simulink model "quad_CAD_asgsm"  (R2024a)
settings: Solver=ode4  StartTime=0.0  StopTime=60  FixedStep=0.01  RelTol=1e-3
undefined symbols (not defined in the file): F, Light, MIL, smiData, X, Y, Z
libraries: sm_lib x221, nesl_utility x22, dspobslib x9, sharedtransform x6, simulink x3, aerolibutil x2, matrix_library x1, sharedutil x1, robotcorelib x1, aerolibwind2 x1
(part 3 of 7)

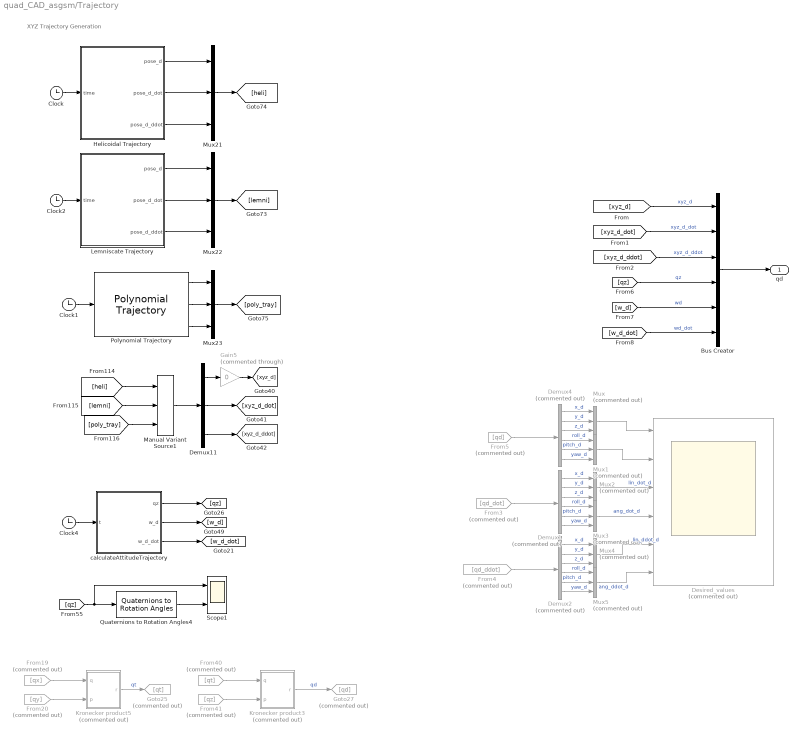
== system quad_CAD_asgsm/Trajectory ==
  note: XYZ Trajectory Generation
  Bus Creator : BusCreator  Inputs=6
  Clock{,1..2,4} (4 alike) : Clock
  Demux1 : Demux  Commented=on  Outputs=6
  Demux11 : Demux  Outputs=3
  Demux2 : Demux  Commented=on  Outputs=6
  Demux4 : Demux  Commented=on  Outputs=6
  Desired_values : Scope  Commented=on  NumInputPorts=6
  From19 : From  Commented=on  GotoTag=qx
  From20 : From  Commented=on  GotoTag=qy
  From3 : From  Commented=on  GotoTag=qd_dot
  From4 : From  Commented=on  GotoTag=qd_ddot
  From40 : From  Commented=on  GotoTag=qt
  From41 : From  Commented=on  GotoTag=qz
  From5 : From  Commented=on  GotoTag=qd
  Gain5 : Gain  Commented=through  Gain=0
  Goto25 : Goto  Commented=on  GotoTag=qt
  Goto27 : Goto  Commented=on  GotoTag=qd
  Helicoidal Trajectory : MATLAB Function  TreatAsAtomicUnit=on
  Kronecker product3 : Subsystem  Commented=on
  Kronecker product5 : Subsystem  Commented=on
  Lemniscate Trajectory : MATLAB Function  TreatAsAtomicUnit=on
  Manual Variant Source1 : simulink/Signal Routing/Manual Variant Source  NumChoices=3  LabelModeActiveChoice=V_3
  Mux{,1..5} (6 alike) : Mux  Commented=on  Inputs=3
  Mux21 : Mux  Inputs=3
  Mux22 : Mux  Inputs=3
  Mux23 : Mux  Inputs=3
  Polynomial Trajectory : robotcorelib/Polynomial Trajectory  WaypointSource=Internal  Waypoints=zeros(3, 6)  TimePoints=[ 0, 12, 24, 36, 48, 60]  TimeInterval=[ 1, 4 ]  Method=Cubic Polynomial  ParameterSource=Internal  VelocityBoundaryCondition=zeros( 3, 6)  AccelerationBoundaryCondition=zeros( 2, 5 )  SimulateUsing=Interpreted execution
  Quaternions to Rotation Angles4 : sharedtransform/Quaternions to Rotation Angles  rotationOrder=ZYX  aMode=aMode
  Scope1 : Scope  NumInputPorts=2
  calculateAttitudeTrajectory : MATLAB Function  TreatAsAtomicUnit=on
  qd : Outport
  wires:
  Demux4/6 -> Mux1/3  "yaw_d"
  Helicoidal Trajectory/2(pose_d_dot) -> Mux21/2
  Demux2/5 -> Mux5/2  "pitch_d"
  Demux4/1 -> Mux/1  "x_d"
  From3/1 -> Demux1/1
  calculateAttitudeTrajectory/3(w_d_dot) -> [w_d_dot]
  [xyz_d_dot] -> Bus Creator/2  "xyz_d_dot"
  Lemniscate Trajectory/1(pose_d) -> Mux22/1
  Bus Creator/1 -> qd/1
  Kronecker product5/1(r) -> Goto25/1  "qt"
  Demux2/6 -> Mux5/3  "yaw_d"
  From20/1 -> Kronecker product5/2(p)
  Demux1/6 -> Mux3/3  "yaw_d"
  Mux1/1 -> Desired_values/2
  From41/1 -> Kronecker product3/2(p)
  From40/1 -> Kronecker product3/1(q)
  Demux11/2 -> [xyz_d_dot]
  Lemniscate Trajectory/3(pose_d_ddot) -> Mux22/3
  Mux/1 -> Desired_values/1
  Lemniscate Trajectory/2(pose_d_dot) -> Mux22/2
  [lemni] -> Manual Variant Source1/2
  Gain5/1 -> [xyz_d]
  From19/1 -> Kronecker product5/1(q)
  Demux4/2 -> Mux/2  "y_d"
  Mux2/1 -> Desired_values/3  "lin_dot_d"
  [xyz_d] -> Bus Creator/1  "xyz_d"
  Demux4/5 -> Mux1/2  "pitch_d"
  Polynomial Trajectory/2 -> Mux23/2
  Helicoidal Trajectory/3(pose_d_ddot) -> Mux21/3
  [heli] -> Manual Variant Source1/1
  [w_d] -> Bus Creator/5  "wd"
  Polynomial Trajectory/3 -> Mux23/3
  Clock/1 -> Helicoidal Trajectory/1(time)
  calculateAttitudeTrajectory/2(w_d) -> [w_d]
  Demux2/1 -> Mux4/1  "x_d"
  [qz] -> Bus Creator/4  "qz"
  Clock4/1 -> calculateAttitudeTrajectory/1(t)
  Mux22/1 -> [lemni]
  [qz] -> Scope1/1, Quaternions to Rotation Angles4/1
  Clock2/1 -> Lemniscate Trajectory/1(time)
  Polynomial Trajectory/1 -> Mux23/1
  calculateAttitudeTrajectory/1(qz) -> [qz]
  Mux21/1 -> [heli]
  Demux4/3 -> Mux/3  "z_d"
  Demux2/4 -> Mux5/1  "roll_d"
  Mux3/1 -> Desired_values/4  "ang_dot_d"
  Mux4/1 -> Desired_values/5  "lin_ddot_d"
  Demux4/4 -> Mux1/1  "roll_d"
  Demux1/1 -> Mux2/1  "x_d"
  Demux1/2 -> Mux2/2  "y_d"
  [xyz_d_ddot] -> Bus Creator/3  "xyz_d_ddot"
  Demux2/3 -> Mux4/3  "z_d"
  From4/1 -> Demux2/1
  [w_d_dot] -> Bus Creator/6  "wd_dot"
  Mux5/1 -> Desired_values/6  "ang_ddot_d"
  Demux11/1 -> Gain5/1
  [poly_tray] -> Manual Variant Source1/3
  From5/1 -> Demux4/1
  Clock1/1 -> Polynomial Trajectory/1
  Kronecker product3/1(r) -> Goto27/1  "qd"
  Quaternions to Rotation Angles4/1 -> Scope1/2
  Helicoidal Trajectory/1(pose_d) -> Mux21/1
  Mux23/1 -> [poly_tray]
  Demux1/3 -> Mux2/3  "z_d"
  Demux1/4 -> Mux3/1  "roll_d"
  Manual Variant Source1/1 -> Demux11/1
  Demux11/3 -> [xyz_d_ddot]
  Demux1/5 -> Mux3/2  "pitch_d"
  Demux2/2 -> Mux4/2  "y_d"

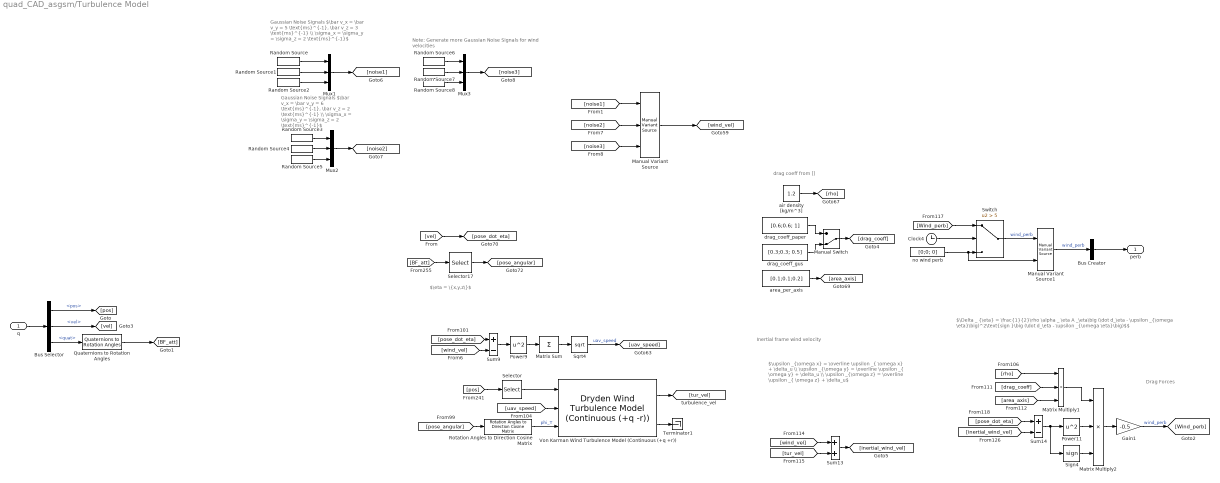
== system quad_CAD_asgsm/Turbulence Model ==
  note: Note: Generate more Gaussian Noise Signals
      | for wind velocities
  note: $\Delta _ {\eta} = \frac{1}{2}\rho \alpha _ \eta A _\eta\big (\dot d_\eta - \upsilon _{\omega \eta}\big)^2\text{sign }\big (\dot d_\eta - \upsilon _{\omega \eta}\big)$$
  note: $\upsilon _{\omega x} = \overline \upsilon _{ \omega x} + \delta_u \\ \upsilon _{\omega y} = \overline \upsilon _{ \omega y} + \delta_u \\ \upsilon _{\omega z} = \overline \upsilon _{ \omega z} + \delta_u$
  note: drag coeff from []
  note: Drag Forces
  note: Inertial frame wind velocity
  note: $\eta = \{x,y,z\}$
  note: Gaussian Noise Signals
      | $\bar v_x = \bar v_y = 6 \text{ms}^{-1}, \bar v_z = 2 \text{ms}^{-1} \\ \sigma_x = \sigma_y = \sigma_z = 2 \text{ms}^{-1}$
  note: Gaussian Noise Signals
      | $\bar v_x = \bar v_y = 5 \text{ms}^{-1}, \bar v_z = 3 \text{ms}^{-1} \\ \sigma_x = \sigma_y = \sigma_z = 2 \text{ms}^{-1}$
  q : Inport
  Bus Creator : BusCreator  Inputs=1
  Bus Selector : BusSelector  OutputSignals=pos,vel,quat
  Clock4 : Clock
  Gain1 : Gain  Gain=-0.5
  Manual Variant Source : simulink/Signal Routing/Manual Variant Source  NumChoices=3  LabelModeActiveChoice=V_1
  Manual Variant Source1 : simulink/Signal Routing/Manual Variant Source  NumChoices=2  LabelModeActiveChoice=V_1
  Manual Switch : ManualSwitch  CurrentSetting=0
  Matrix Sum : Sum  Inputs=+
  Matrix Multiply1 : Product  Inputs=3
  Matrix Multiply2 : Product  Inputs=3
  Mux1 : Mux  Inputs=3
  Mux2 : Mux  Inputs=3
  Mux3 : Mux  Inputs=3
  Power11 : Math  Operator=square
  Power9 : Math  Operator=square
  Quaternions to Rotation Angles : sharedtransform/Quaternions to Rotation Angles  rotationOrder=ZYX  aMode=aMode
  Random Source : dspobslib/Random Source  SrcType=Gaussian  NormMethod=Ziggurat  CltLength=12  MinVal=0  MaxVal=1  MeanVal=5  VarVal=2  RepMode=Not repeatable  rawSeed=1  IsInherit=off  SampMode=Discrete  SampTime=1  SampFrame=1  DataType=Double  OutComplex=Real  OutputFrames=off
  Random Source1 : dspobslib/Random Source  SrcType=Gaussian  NormMethod=Ziggurat  CltLength=12  MinVal=0  MaxVal=1  MeanVal=5  VarVal=2  RepMode=Not repeatable  rawSeed=1  IsInherit=off  SampMode=Discrete  SampTime=1  SampFrame=1  DataType=Double  OutComplex=Real  OutputFrames=off
  Random Source2 : dspobslib/Random Source  SrcType=Gaussian  NormMethod=Ziggurat  CltLength=12  MinVal=0  MaxVal=1  MeanVal=3  VarVal=2  RepMode=Not repeatable  rawSeed=1  IsInherit=off  SampMode=Discrete  SampTime=1  SampFrame=1  DataType=Double  OutComplex=Real  OutputFrames=off
  Random Source{3..4,6..7} (4 alike) : dspobslib/Random Source  SrcType=Gaussian  NormMethod=Ziggurat  CltLength=12  MinVal=0  MaxVal=1  MeanVal=6  VarVal=2  RepMode=Not repeatable  rawSeed=1  IsInherit=off  SampMode=Discrete  SampTime=1  SampFrame=1  DataType=Double  OutComplex=Real  OutputFrames=off
  Random Source5 : dspobslib/Random Source  SrcType=Gaussian  NormMethod=Ziggurat  CltLength=12  MinVal=0  MaxVal=1  MeanVal=2  VarVal=2  RepMode=Not repeatable  rawSeed=1  IsInherit=off  SampMode=Discrete  SampTime=1  SampFrame=1  DataType=Double  OutComplex=Real  OutputFrames=off
  Random Source8 : dspobslib/Random Source  SrcType=Gaussian  NormMethod=Ziggurat  CltLength=12  MinVal=0  MaxVal=1  MeanVal=2  VarVal=2  RepMode=Not repeatable  rawSeed=1  IsInherit=off  SampMode=Discrete  SampTime=1  SampFrame=1  DataType=Double  OutComplex=Real  OutputFrames=off
  Rotation Angles to Direction Cosine Matrix : sharedtransform/Rotation Angles to Direction Cosine Matrix  rotationOrder=XYZ  aMode=aMode
  Selector : Selector  InputPortWidth=3  IndexOptions=Index vector (dialog)  Indices=[3]  OutputSizes=1
  Selector17 : Selector  InputPortWidth=3  IndexOptions=Index vector (dialog)  Indices=[3 2 1]  OutputSizes=1
  Sign4 : Signum
  Sqrt4 : Sqrt
  Sum13 : Sum
  Sum14 : Sum  Inputs=+-
  Sum9 : Sum  Inputs=+-
  Switch : Switch  Criteria=u2 > Threshold  Threshold=5  SaturateOnIntegerOverflow=off  InputSameDT=off
  Terminator1 : Terminator
  Von Karman Wind Turbulence Model (Continuous (+q +r)) : aerolibwind2/Dryden Wind Turbulence Model  (Continuous (+q -r))  units=Metric (MKS)  spec=MIL-F-8785C  model=Continuous Von Karman (+q -r)  W20=15  Wdeg=0  TurbProb=10^-2 - Light  L_high=762  Wingspan=10  ts=0.1  Seed=[23341 23342 23343 23344]  T_on=on
      settings: LibrarySourceBlock=|
      | aerolibwind2/Von Karman Wind Turbulence Model
      | (Continuous (+q +r))
  air density [kg/m^3] : Constant  Value=1.2
  area_per_axis : Constant  Value=[0.1;0.1;0.2]
  drag_coeff_gus : Constant  Value=[0.3;0.3; 0.5]
  drag_coeff_paper : Constant  Value=[0.6;0.6; 1]
  no wind perb : Constant  Value=[0;0; 0]
  perb : Outport
  wires:
  [rho] -> Matrix Multiply1/1
  [drag_coeff] -> Matrix Multiply1/2
  Von Karman Wind Turbulence Model (Continuous (+q +r))/2 -> Terminator1/1
  area_per_axis/1 -> [area_axis]
  [pose_dot_eta] -> Sum14/1
  Von Karman Wind Turbulence Model (Continuous (+q +r))/1 -> [tur_vel]
  [wind_vel] -> Sum9/2
  Selector17/1 -> [pose_angular]
  Matrix Multiply1/1 -> Matrix Multiply2/1
  Sign4/1 -> Matrix Multiply2/3
  [uav_speed] -> Von Karman Wind Turbulence Model (Continuous (+q +r))/2
  Power9/1 -> Matrix Sum/1
  Sqrt4/1 -> [uav_speed]  "uav_speed"
  Gain1/1 -> [Wind_perb]  "wind_perb"
  Sum9/1 -> Power9/1
  air density [kg/m^3]/1 -> [rho]
  Clock4/1 -> Switch/2
  [pose_dot_eta] -> Sum9/1
  Rotation Angles to Direction Cosine Matrix/1 -> Von Karman Wind Turbulence Model (Continuous (+q +r))/3  "phi_T"
  [tur_vel] -> Sum13/2
  Sum14/1 -> Sign4/1, Power11/1
  no wind perb/1 -> Manual Variant Source1/2, Switch/3
  drag_coeff_gus/1 -> Manual Switch/2
  Switch/1 -> Manual Variant Source1/1  "wind_perb"
  [area_axis] -> Matrix Multiply1/3
  Manual Switch/1 -> [drag_coeff]
  Selector/1 -> Von Karman Wind Turbulence Model (Continuous (+q +r))/1
  [pose_angular] -> Rotation Angles to Direction Cosine Matrix/1
  [inertial_wind_vel] -> Sum14/2
  Matrix Multiply2/1 -> Gain1/1
  drag_coeff_paper/1 -> Manual Switch/1
  Power11/1 -> Matrix Multiply2/2
  Matrix Sum/1 -> Sqrt4/1
  Sum13/1 -> [inertial_wind_vel]
  [Wind_perb] -> Switch/1
  [wind_vel] -> Sum13/1
  Bus Creator/1 -> perb/1
  [BF_att] -> Selector17/1
  [pos] -> Selector/1
  q/1 -> Bus Selector/1
  Bus Selector/1 -> [pos]  "<pos>"
  Bus Selector/3 -> Quaternions to Rotation Angles/1  "<quat>"
  Bus Selector/2 -> [vel]  "<vel>"
  [vel] -> [pose_dot_eta]
  Mux2/1 -> [noise2]
  Random Source5/1 -> Mux2/3
  Random Source/1 -> Mux1/1
  Mux1/1 -> [noise1]
  Random Source2/1 -> Mux1/3
  Random Source4/1 -> Mux2/2
  Random Source3/1 -> Mux2/1
  [noise2] -> Manual Variant Source/2
  Manual Variant Source/1 -> [wind_vel]
  Random Source1/1 -> Mux1/2
  [noise1] -> Manual Variant Source/1
  [noise3] -> Manual Variant Source/3
  Mux3/1 -> [noise3]
  Random Source7/1 -> Mux3/2
  Random Source6/1 -> Mux3/1
  Random Source8/1 -> Mux3/3
  Manual Variant Source1/1 -> Bus Creator/1  "wind_perb"
  Quaternions to Rotation Angles/1 -> [BF_att]

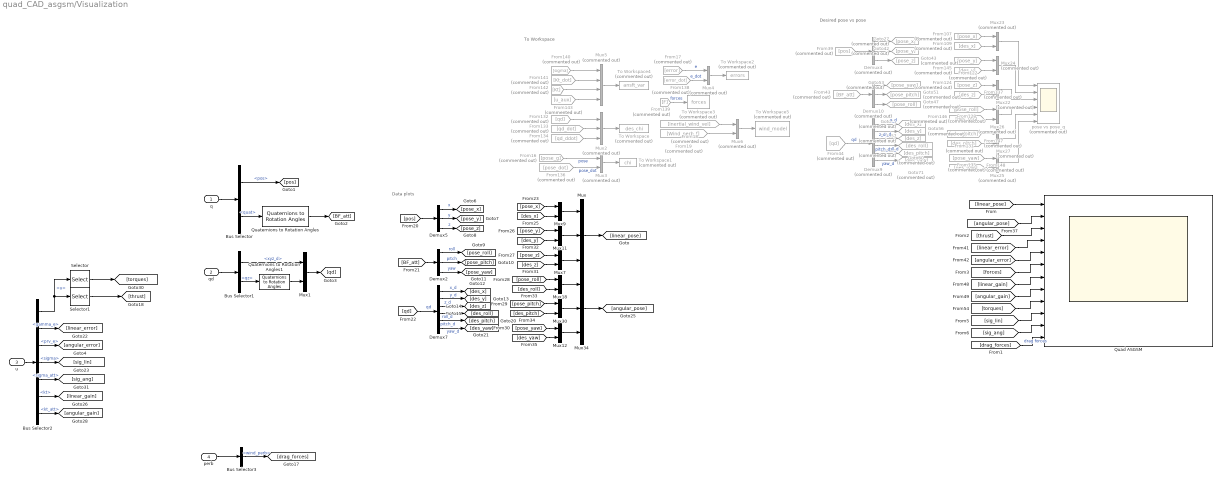
== system quad_CAD_asgsm/Visualization ==
  note: Desired pose vs pose
  note: Data plots
  note: To Workspace
  q : Inport
  qd : Inport  Port=2
  u : Inport  Port=3
  perb : Inport  Port=4
  Bus Selector : BusSelector  OutputSignals=pos,quat
  Bus Selector1 : BusSelector  OutputSignals=xyz_d,qz
  Bus Selector2 : BusSelector  OutputSignals=u,gamma_e,prv_e,sigma,sigma_att,kt,kt_att
  Bus Selector3 : BusSelector  OutputSignals=wind_perb
  Demux10 : Demux  Commented=on  Outputs=3
  Demux2 : Demux  Outputs=3
  Demux4 : Demux  Commented=on  Outputs=3
  Demux5 : Demux  Outputs=3
  Demux7 : Demux  Outputs=6
  Demux9 : Demux  Commented=on  Outputs=6
  From107 : From  Commented=on  GotoTag=pose_x
  From109 : From  Commented=on  GotoTag=des_x
  From122 : From  Commented=on  GotoTag=pose_y
  From124 : From  Commented=on  GotoTag=pose_z
  From128 : From  Commented=on  GotoTag=pose_roll
  From131 : From  Commented=on  GotoTag=pose_pitch
  From132 : From  Commented=on  GotoTag=qd
  From133 : From  Commented=on  GotoTag=qd_dot
  From134 : From  Commented=on  GotoTag=qd_ddot
  From135 : From  Commented=on  GotoTag=pose_yaw
  From136 : From  Commented=on  GotoTag=pose_dot
  From137 : From  Commented=on  GotoTag=des_z
  From138 : From  Commented=on  GotoTag=error_dot
  From139 : From  Commented=on  GotoTag=F
  From140 : From  Commented=on  GotoTag=sigma
  From141 : From  Commented=on  GotoTag=Kt_dot
  From142 : From  Commented=on  GotoTag=Kt
  From143 : From  Commented=on  GotoTag=u_aux
  From145 : From  Commented=on  GotoTag=des_y
  From146 : From  Commented=on  GotoTag=des_roll
  From147 : From  Commented=on  GotoTag=des_pitch
  From148 : From  Commented=on  GotoTag=des_yaw
  From16 : From  Commented=on  GotoTag=pose_g
  From17 : From  Commented=on  GotoTag=error
  From18 : From  Commented=on  GotoTag=inertial_wind_vel
  From19 : From  Commented=on  GotoTag=Wind_perb_f  TagVisibility=global
  From39 : From  Commented=on  GotoTag=pos
  From43 : From  Commented=on  GotoTag=BF_att
  From44 : From  Commented=on  GotoTag=qd
  Goto27 : Goto  Commented=on  GotoTag=pose_x
  Goto42 : Goto  Commented=on  GotoTag=pose_y
  Goto43 : Goto  Commented=on  GotoTag=pose_z
  Goto47 : Goto  Commented=on  GotoTag=pose_roll
  Goto51 : Goto  Commented=on  GotoTag=pose_pitch
  Goto53 : Goto  Commented=on  GotoTag=pose_yaw
  Goto55 : Goto  Commented=on  GotoTag=des_x
  Goto56 : Goto  Commented=on  GotoTag=des_y
  Goto57 : Goto  Commented=on  GotoTag=des_z
  Goto60 : Goto  Commented=on  GotoTag=des_roll
  Goto68 : Goto  Commented=on  GotoTag=des_pitch
  Goto71 : Goto  Commented=on  GotoTag=des_yaw
  Mux : Mux  Inputs=3
  Mux{1,7,9,11..12,18,30} (7 alike) : Mux  Inputs=2
  Mux2 : Mux  Commented=on  Inputs=3
  Mux{3..4,6,22..27} (9 alike) : Mux  Commented=on  Inputs=2
  Mux34 : Mux  Inputs=3
  Mux5 : Mux  Commented=on
  Quad ASGSM : Scope  NumInputPorts=12
  Quaternions to Rotation Angles : sharedtransform/Quaternions to Rotation Angles  rotationOrder=XYZ  aMode=aMode
  Quaternions to Rotation Angles1 : sharedtransform/Quaternions to Rotation Angles  rotationOrder=XYZ  aMode=aMode
  Selector : Selector  InputPortWidth=4  IndexOptions=Index vector (dialog)  Indices=[1:3]  OutputSizes=1
  Selector1 : Selector  InputPortWidth=4  IndexOptions=Index vector (dialog)  Indices=[4]  OutputSizes=1
  To Workspace : ToWorkspace  Commented=on  VariableName=des_chi  SaveFormat=Structure With Time  SampleTime=-1
  To Workspace1 : ToWorkspace  Commented=on  VariableName=chi  SaveFormat=Structure With Time  SampleTime=-1
  To Workspace2 : ToWorkspace  Commented=on  VariableName=errors  SaveFormat=Structure With Time  SampleTime=-1
  To Workspace3 : ToWorkspace  Commented=on  VariableName=forces  SaveFormat=Structure With Time  SampleTime=-1
  To Workspace4 : ToWorkspace  Commented=on  VariableName=ansft_var  SaveFormat=Structure With Time  SampleTime=-1
  To Workspace5 : ToWorkspace  Commented=on  VariableName=wind_model  SaveFormat=Structure With Time  SampleTime=-1
  pose vs pose_q : Scope  Commented=on  NumInputPorts=6
  wires:
  Mux/1 -> [linear_pose]
  Mux6/1 -> To Workspace5/1
  Mux9/1 -> Mux/1
  From128/1 -> Mux26/1
  Demux4/1 -> Goto27/1
  Demux7/5 -> [des_pitch]  "pitch_d"
  From135/1 -> Mux25/1
  [linear_error] -> Quad ASGSM/4
  [angular_error] -> Quad ASGSM/5
  From132/1 -> Mux2/1
  Mux11/1 -> Mux/2
  Demux4/3 -> Goto43/1
  Demux5/1 -> [pose_x]  "x"
  Demux10/1 -> Goto53/1
  Demux10/3 -> Goto47/1
  Mux3/1 -> To Workspace1/1
  Demux5/3 -> [pose_z]  "z"
  From148/1 -> Mux25/2
  Demux9/6 -> Goto71/1  "yaw_d"
  [BF_att] -> Demux2/1
  Mux23/1 -> pose vs pose_q/1
  Demux9/2 -> Goto56/1  "y_d"
  Demux7/2 -> [des_y]  "y_d"
  Demux5/2 -> [pose_y]  "y"
  From16/1 -> Mux3/1  "pose"
  [pose_pitch] -> Mux30/1
  [pose_y] -> Mux11/1
  From44/1 -> Demux9/1  "qd"
  Demux7/3 -> [des_z]  "z_d"
  [angular_gain] -> Quad ASGSM/8
  From133/1 -> Mux2/2
  [des_pitch] -> Mux30/2
  Mux5/1 -> To Workspace4/1
  [linear_gain] -> Quad ASGSM/7
  Mux2/1 -> To Workspace/1
  [des_roll] -> Mux18/2
  From43/1 -> Demux10/1
  Mux22/1 -> pose vs pose_q/3
  Mux26/1 -> pose vs pose_q/4
  Mux24/1 -> pose vs pose_q/2
  From109/1 -> Mux23/2
  Demux7/4 -> [des_roll]  "roll_d"
  Demux9/4 -> Goto60/1  "roll_d"
  From122/1 -> Mux24/1
  [des_yaw] -> Mux12/2
  From139/1 -> To Workspace3/1  "forces"
  [angular_pose] -> Quad ASGSM/2
  Demux9/3 -> Goto57/1  "z_d"
  From124/1 -> Mux22/1
  Demux7/1 -> [des_x]  "x_d"
  From138/1 -> Mux4/2  "e_dot"
  [pose_yaw] -> Mux12/1
  From39/1 -> Demux4/1
  From137/1 -> Mux22/2
  Mux12/1 -> Mux34/3
  From131/1 -> Mux27/1
  [des_x] -> Mux9/2
  [linear_pose] -> Quad ASGSM/1
  Demux9/1 -> Goto55/1  "x_d"
  [pos] -> Demux5/1
  From18/1 -> Mux6/1
  From141/1 -> Mux5/2
  Mux7/1 -> Mux/3
  From145/1 -> Mux24/2
  Demux9/5 -> Goto68/1  "pitch_d"
  From17/1 -> Mux4/1  "e"
  Mux34/1 -> [angular_pose]
  [pose_x] -> Mux9/1
  Demux10/2 -> Goto51/1
  [pose_roll] -> Mux18/1
  [pose_z] -> Mux7/1
  Mux30/1 -> Mux34/2
  [des_y] -> Mux11/2
  Demux7/6 -> [des_yaw]  "yaw_d"
  Mux4/1 -> To Workspace2/1
  From19/1 -> Mux6/2
  From134/1 -> Mux2/3
  Mux18/1 -> Mux34/1
  Demux4/2 -> Goto42/1
  [qd] -> Demux7/1  "qd"
  From143/1 -> Mux5/4
  From146/1 -> Mux26/2
  Mux27/1 -> pose vs pose_q/5
  [des_z] -> Mux7/2
  From147/1 -> Mux27/2
  From142/1 -> Mux5/3
  From140/1 -> Mux5/1
  From136/1 -> Mux3/2  "pose_dot"
  From107/1 -> Mux23/1
  Mux25/1 -> pose vs pose_q/6
  q/1 -> Bus Selector/1
  Bus Selector/1 -> [pos]  "<pos>"
  Bus Selector/2 -> Quaternions to Rotation Angles/1  "<quat>"
  qd/1 -> Bus Selector1/1
  Bus Selector1/1 -> Mux1/1  "<xyz_d>"
  u/1 -> Bus Selector2/1
  perb/1 -> Bus Selector3/1
  Bus Selector3/1 -> [drag_forces]  "<wind_perb>"
  [thrust] -> Quad ASGSM/3
  [forces] -> Quad ASGSM/6
  [torques] -> Quad ASGSM/9
  [drag_forces] -> Quad ASGSM/12  "drag forces"
  [sig_lin] -> Quad ASGSM/10
  [sig_ang] -> Quad ASGSM/11
  Demux2/2 -> [pose_pitch]  "pitch"
  Demux2/3 -> [pose_yaw]  "yaw"
  Demux2/1 -> [pose_roll]  "roll"
  Quaternions to Rotation Angles/1 -> [BF_att]
  Bus Selector2/1 -> Selector1/1, Selector/1  "<u>"
  Selector/1 -> [torques]
  Selector1/1 -> [thrust]
  Bus Selector2/5 -> [sig_ang]  "<sigma_att>"
  Bus Selector2/7 -> [angular_gain]  "<kt_att>"
  Bus Selector2/6 -> [linear_gain]  "<kt>"
  Bus Selector2/4 -> [sig_lin]  "<sigma>"
  Bus Selector2/3 -> [angular_error]  "<prv_e>"
  Bus Selector2/2 -> [linear_error]  "<gamma_e>"
  Bus Selector1/2 -> Quaternions to Rotation Angles1/1  "<qz>"
  Quaternions to Rotation Angles1/1 -> Mux1/2
  Mux1/1 -> [qd]

== system quad_CAD_asgsm/Controller/Attitude_Alignment ==
  nu : Inport
  nz : Inport  Port=2
  Scope : Scope  NumInputPorts=2
  attitude_alignment : MATLAB Function  TreatAsAtomicUnit=on
  qt : Outport
  wires:
  attitude_alignment/1(qt) -> qt/1
  nz/1 -> attitude_alignment/2("nz ")
  nu/1 -> attitude_alignment/1(u)
  attitude_alignment/2(nz) -> Scope/1
  attitude_alignment/3(nu) -> Scope/2

== system quad_CAD_asgsm/Controller/Kronecker product3 ==
  q : Inport
  p : Inport  Port=2
  Kronecker_product : MATLAB Function  TreatAsAtomicUnit=on
  r : Outport
  wires:
  q/1 -> Kronecker_product/1(q)
  p/1 -> Kronecker_product/2(p)
  Kronecker_product/1(r) -> r/1

== system quad_CAD_asgsm/Controller/Kronecker product4 ==
  q : Inport
  p : Inport  Port=2
  Kronecker_product : MATLAB Function  TreatAsAtomicUnit=on
  r : Outport
  wires:
  q/1 -> Kronecker_product/1(q)
  p/1 -> Kronecker_product/2(p)
  Kronecker_product/1(r) -> r/1

== system quad_CAD_asgsm/Controller/Subsystem1 ==
  q : Inport
  MATLAB Function : MATLAB Function  TreatAsAtomicUnit=on
  lnq : Outport
  wires:
  MATLAB Function/1(lnq) -> lnq/1
  q/1 -> MATLAB Function/1(q)

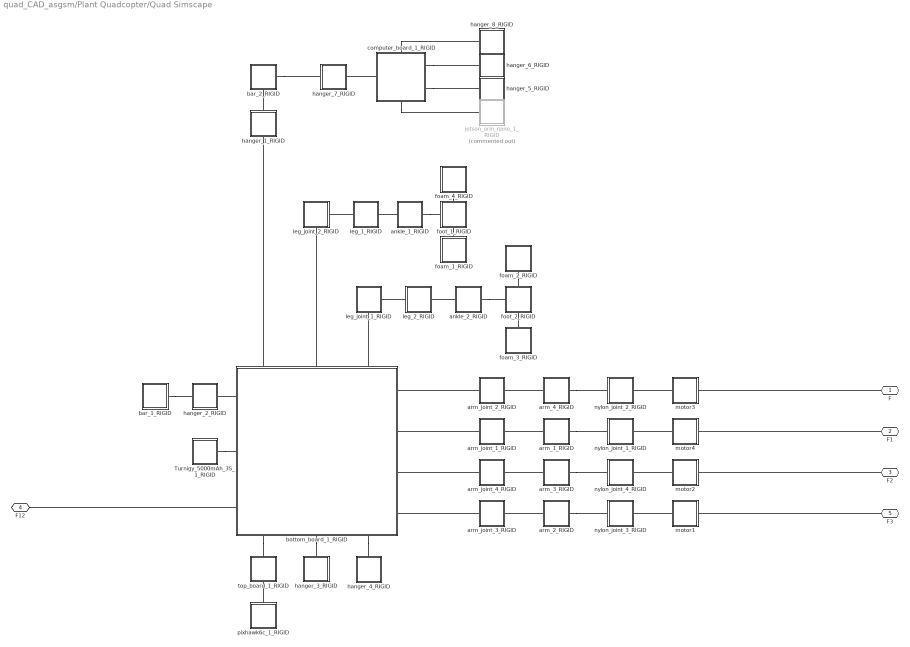
== system quad_CAD_asgsm/Plant Quadcopter/Quad Simscape ==
  Turnigy_5000mAh_3S_1_RIGID : Subsystem
  ankle_1_RIGID : Subsystem
  ankle_2_RIGID : Subsystem
  arm_1_RIGID : Subsystem
  arm_2_RIGID : Subsystem
  arm_3_RIGID : Subsystem
  arm_4_RIGID : Subsystem
  arm_joint_1_RIGID : Subsystem
  arm_joint_2_RIGID : Subsystem
  arm_joint_3_RIGID : Subsystem
  arm_joint_4_RIGID : Subsystem
  bar_1_RIGID : Subsystem
  bar_2_RIGID : Subsystem
      settings: PortSchema="{\"entries\":[{\"content\":{\"sides\":[{\"content\":{},\"type\":\"ConnectorPlacement.EquallySpacedRectSide\",\"uuid\":\"e4c68bcb-f3fe-4aba-8bbb-748bf6c2ba1e\"},{\"content\":{\"connectorIds\":[\"RConn1\"],\"side\":\"RIGHT\"},\"type\":\"ConnectorPlacement.EquallySpacedRectSide\",\"uuid\":\"1338b84e-cb3b-43ed-b934-4b64495642c6\"},{\"content\":{\"side\":\"TOP\"},\"type\":\"ConnectorPlacement.EquallySpacedRectSide\",\"uuid\":\"c07eb51d-104f-4d2f-bffb-19c5e8e904cd\"},{\"content\":{\"connectorIds\":[\"RConn2\"],\"side\":\"BOTTOM\"},\"type\":\"ConnectorPlacement.EquallySpacedRectSide\",\"uuid\":\"9f3520f2-c2cf-4d2b-85d9-f0e92fcce62d\"}]},\"type\":\"ConnectorPlacement.EquallySpacedConnector\",\"uuid\":\"66267511-5957-447d-be6d-58b2f28344a3\"}],\"packageUris\":[\"http://schema.mathworks.com/mf0/Connector/R2020b\"],\"version\":\"1.0\"}"
  bottom_board_1_RIGID : Subsystem
      settings: PortSchema="{\"entries\":[{\"content\":{\"sides\":[{\"content\":{\"connectorIds\":[\"LConn1\",\"LConn2\",\"LConn3\"]},\"type\":\"ConnectorPlacement.EquallySpacedRectSide\",\"uuid\":\"9aceb689-13c3-4410-a12b-a205fc5c5e29\"},{\"content\":{\"connectorIds\":[\"RConn1\",\"RConn2\",\"RConn3\",\"RConn4\"],\"side\":\"RIGHT\"},\"type\":\"ConnectorPlacement.EquallySpacedRectSide\",\"uuid\":\"62657ca3-c014-471d-8baa-8f5757c474c2\"},{\"content\":{\"connectorIds\":[\"LConn4\",\"LConn5\",\"LConn6\"],\"side\":\"TOP\"},\"type\":\"ConnectorPlacement.EquallySpacedRectSide\",\"uuid\":\"f572a818-8233-41db-820d-2371a42ad6c7\"},{\"content\":{\"connectorIds\":[\"RConn5\",\"RConn6\",\"RConn7\"],\"side\":\"BOTTOM\"},\"type\":\"ConnectorPlacement.EquallySpacedRectSide\",\"uuid\":\"f4e3c856-449b-45f8-8e8a-d1faf7fe0ed6\"}]},\"type\":\"ConnectorPlacement.EquallySpacedConnector\",\"uuid\":\"18325c75-42ae-41d5-ba8b-a65f9cc18b57\"}],\"packageUris\":[\"http://schema.mathworks.com/mf0/Connector/R2020b\"],\"version\":\"1.0\"}"
  computer_board_1_RIGID : Subsystem
      settings: PortSchema="{\"entries\":[{\"content\":{\"sides\":[{\"content\":{\"connectorIds\":[\"LConn1\"]},\"type\":\"ConnectorPlacement.EquallySpacedRectSide\",\"uuid\":\"45520a5c-9755-44f8-961d-1edc3bf3f9b3\"},{\"content\":{\"connectorIds\":[\"RConn1\",\"RConn2\"],\"side\":\"RIGHT\"},\"type\":\"ConnectorPlacement.EquallySpacedRectSide\",\"uuid\":\"004a0d01-52c5-40e4-bd02-7a89b4d4e543\"},{\"content\":{\"connectorIds\":[\"LConn2\"],\"side\":\"TOP\"},\"type\":\"ConnectorPlacement.EquallySpacedRectSide\",\"uuid\":\"74e8819f-1d4d-4a14-976c-d3b18c4e091d\"},{\"content\":{\"connectorIds\":[\"RConn3\"],\"side\":\"BOTTOM\"},\"type\":\"ConnectorPlacement.EquallySpacedRectSide\",\"uuid\":\"f917d1f0-d232-4281-b426-7e15d7693ef0\"}]},\"type\":\"ConnectorPlacement.EquallySpacedConnector\",\"uuid\":\"e479e9d8-600b-48d5-99b2-6391ef29c8cc\"}],\"packageUris\":[\"http://schema.mathworks.com/mf0/Connector/R2020b\"],\"version\":\"1.0\"}"
  foam_1_RIGID : Subsystem
      settings: PortSchema="{\"entries\":[{\"content\":{\"sides\":[{\"content\":{},\"type\":\"ConnectorPlacement.EquallySpacedRectSide\",\"uuid\":\"7acb360a-1230-4e27-92b8-6b3184352f22\"},{\"content\":{\"side\":\"RIGHT\"},\"type\":\"ConnectorPlacement.EquallySpacedRectSide\",\"uuid\":\"8c89d56c-1eb2-4c7c-8666-e0d9ca480c9b\"},{\"content\":{\"connectorIds\":[\"LConn1\"],\"side\":\"TOP\"},\"type\":\"ConnectorPlacement.EquallySpacedRectSide\",\"uuid\":\"50379f80-a646-4b72-9568-e30937a88a17\"}]},\"type\":\"ConnectorPlacement.EquallySpacedConnector\",\"uuid\":\"0fd64392-f5bf-42bb-9262-b488cfdbbdbf\"}],\"packageUris\":[\"http://schema.mathworks.com/mf0/Connector/R2020b\"],\"version\":\"1.0\"}"
  foam_2_RIGID : Subsystem
      settings: PortSchema="{\"entries\":[{\"content\":{\"sides\":[{\"content\":{},\"type\":\"ConnectorPlacement.EquallySpacedRectSide\",\"uuid\":\"7acb360a-1230-4e27-92b8-6b3184352f22\"},{\"content\":{\"side\":\"RIGHT\"},\"type\":\"ConnectorPlacement.EquallySpacedRectSide\",\"uuid\":\"8c89d56c-1eb2-4c7c-8666-e0d9ca480c9b\"},{\"content\":{\"side\":\"TOP\"},\"type\":\"ConnectorPlacement.EquallySpacedRectSide\",\"uuid\":\"50379f80-a646-4b72-9568-e30937a88a17\"},{\"content\":{\"connectorIds\":[\"RConn1\"],\"side\":\"BOTTOM\"},\"type\":\"ConnectorPlacement.EquallySpacedRectSide\",\"uuid\":\"d189d42a-5809-41f4-8819-94bfeb6d4069\"}]},\"type\":\"ConnectorPlacement.EquallySpacedConnector\",\"uuid\":\"0fd64392-f5bf-42bb-9262-b488cfdbbdbf\"}],\"packageUris\":[\"http://schema.mathworks.com/mf0/Connector/R2020b\"],\"version\":\"1.0\"}"
  foam_3_RIGID : Subsystem
      settings: PortSchema="{\"entries\":[{\"content\":{\"sides\":[{\"content\":{},\"type\":\"ConnectorPlacement.EquallySpacedRectSide\",\"uuid\":\"7acb360a-1230-4e27-92b8-6b3184352f22\"},{\"content\":{\"side\":\"RIGHT\"},\"type\":\"ConnectorPlacement.EquallySpacedRectSide\",\"uuid\":\"8c89d56c-1eb2-4c7c-8666-e0d9ca480c9b\"},{\"content\":{\"connectorIds\":[\"LConn1\"],\"side\":\"TOP\"},\"type\":\"ConnectorPlacement.EquallySpacedRectSide\",\"uuid\":\"50379f80-a646-4b72-9568-e30937a88a17\"}]},\"type\":\"ConnectorPlacement.EquallySpacedConnector\",\"uuid\":\"0fd64392-f5bf-42bb-9262-b488cfdbbdbf\"}],\"packageUris\":[\"http://schema.mathworks.com/mf0/Connector/R2020b\"],\"version\":\"1.0\"}"
  foam_4_RIGID : Subsystem
      settings: PortSchema="{\"entries\":[{\"content\":{\"sides\":[{\"content\":{},\"type\":\"ConnectorPlacement.EquallySpacedRectSide\",\"uuid\":\"7acb360a-1230-4e27-92b8-6b3184352f22\"},{\"content\":{\"side\":\"RIGHT\"},\"type\":\"ConnectorPlacement.EquallySpacedRectSide\",\"uuid\":\"8c89d56c-1eb2-4c7c-8666-e0d9ca480c9b\"},{\"content\":{\"side\":\"TOP\"},\"type\":\"ConnectorPlacement.EquallySpacedRectSide\",\"uuid\":\"50379f80-a646-4b72-9568-e30937a88a17\"},{\"content\":{\"connectorIds\":[\"RConn1\"],\"side\":\"BOTTOM\"},\"type\":\"ConnectorPlacement.EquallySpacedRectSide\",\"uuid\":\"61179d7d-8587-4b45-83e9-ef742d015af7\"}]},\"type\":\"ConnectorPlacement.EquallySpacedConnector\",\"uuid\":\"0fd64392-f5bf-42bb-9262-b488cfdbbdbf\"}],\"packageUris\":[\"http://schema.mathworks.com/mf0/Connector/R2020b\"],\"version\":\"1.0\"}"
  foot_1_RIGID : Subsystem
      settings: PortSchema="{\"entries\":[{\"content\":{\"sides\":[{\"content\":{\"connectorIds\":[\"LConn1\"]},\"type\":\"ConnectorPlacement.EquallySpacedRectSide\",\"uuid\":\"1a0a0e75-7949-47c0-aa82-9aafb0ed1e2e\"},{\"content\":{\"side\":\"RIGHT\"},\"type\":\"ConnectorPlacement.EquallySpacedRectSide\",\"uuid\":\"0e060f82-3302-4f11-ac21-d67ab89e4ef2\"},{\"content\":{\"connectorIds\":[\"LConn2\"],\"side\":\"TOP\"},\"type\":\"ConnectorPlacement.EquallySpacedRectSide\",\"uuid\":\"ad96bb17-0cf4-450d-994f-a350165fc804\"},{\"content\":{\"connectorIds\":[\"RConn1\"],\"side\":\"BOTTOM\"},\"type\":\"ConnectorPlacement.EquallySpacedRectSide\",\"uuid\":\"8a2458c2-19b1-40d9-b853-3966c5a2e466\"}]},\"type\":\"ConnectorPlacement.EquallySpacedConnector\",\"uuid\":\"96350bdb-8090-4c23-8ad2-2b79d30da548\"}],\"packageUris\":[\"http://schema.mathworks.com/mf0/Connector/R2020b\"],\"version\":\"1.0\"}"
  foot_2_RIGID : Subsystem
      settings: PortSchema="{\"entries\":[{\"content\":{\"sides\":[{\"content\":{\"connectorIds\":[\"LConn1\"]},\"type\":\"ConnectorPlacement.EquallySpacedRectSide\",\"uuid\":\"90fae9e9-5946-4121-8f71-91ba44b64005\"},{\"content\":{\"side\":\"RIGHT\"},\"type\":\"ConnectorPlacement.EquallySpacedRectSide\",\"uuid\":\"04a33310-1d26-4df4-bd9d-6ca1a970af75\"},{\"content\":{\"connectorIds\":[\"LConn2\"],\"side\":\"TOP\"},\"type\":\"ConnectorPlacement.EquallySpacedRectSide\",\"uuid\":\"14cd32c8-c7e5-41fd-a063-8cd06ab2c0c0\"},{\"content\":{\"connectorIds\":[\"RConn1\"],\"side\":\"BOTTOM\"},\"type\":\"ConnectorPlacement.EquallySpacedRectSide\",\"uuid\":\"642c07df-7455-4904-bf06-166e866c6230\"}]},\"type\":\"ConnectorPlacement.EquallySpacedConnector\",\"uuid\":\"e570772a-1e43-4802-8b93-014d1a113a22\"}],\"packageUris\":[\"http://schema.mathworks.com/mf0/Connector/R2020b\"],\"version\":\"1.0\"}"
  hanger_1_RIGID : Subsystem
      settings: PortSchema="{\"entries\":[{\"content\":{\"sides\":[{\"content\":{},\"type\":\"ConnectorPlacement.EquallySpacedRectSide\",\"uuid\":\"e4c68bcb-f3fe-4aba-8bbb-748bf6c2ba1e\"},{\"content\":{\"side\":\"RIGHT\"},\"type\":\"ConnectorPlacement.EquallySpacedRectSide\",\"uuid\":\"1338b84e-cb3b-43ed-b934-4b64495642c6\"},{\"content\":{\"connectorIds\":[\"LConn1\"],\"side\":\"TOP\"},\"type\":\"ConnectorPlacement.EquallySpacedRectSide\",\"uuid\":\"c07eb51d-104f-4d2f-bffb-19c5e8e904cd\"},{\"content\":{\"connectorIds\":[\"RConn1\"],\"side\":\"BOTTOM\"},\"type\":\"ConnectorPlacement.EquallySpacedRectSide\",\"uuid\":\"84703210-31b9-465b-91d8-89a356e12aaf\"}]},\"type\":\"ConnectorPlacement.EquallySpacedConnector\",\"uuid\":\"66267511-5957-447d-be6d-58b2f28344a3\"}],\"packageUris\":[\"http://schema.mathworks.com/mf0/Connector/R2020b\"],\"version\":\"1.0\"}"
  hanger_2_RIGID : Subsystem
  hanger_3_RIGID : Subsystem
      settings: PortSchema="{\"entries\":[{\"content\":{\"sides\":[{\"content\":{},\"type\":\"ConnectorPlacement.EquallySpacedRectSide\",\"uuid\":\"7acb360a-1230-4e27-92b8-6b3184352f22\"},{\"content\":{\"side\":\"RIGHT\"},\"type\":\"ConnectorPlacement.EquallySpacedRectSide\",\"uuid\":\"8c89d56c-1eb2-4c7c-8666-e0d9ca480c9b\"},{\"content\":{\"connectorIds\":[\"LConn1\"],\"side\":\"TOP\"},\"type\":\"ConnectorPlacement.EquallySpacedRectSide\",\"uuid\":\"50379f80-a646-4b72-9568-e30937a88a17\"}]},\"type\":\"ConnectorPlacement.EquallySpacedConnector\",\"uuid\":\"0fd64392-f5bf-42bb-9262-b488cfdbbdbf\"}],\"packageUris\":[\"http://schema.mathworks.com/mf0/Connector/R2020b\"],\"version\":\"1.0\"}"
  hanger_4_RIGID : Subsystem
      settings: PortSchema="{\"entries\":[{\"content\":{\"sides\":[{\"content\":{},\"type\":\"ConnectorPlacement.EquallySpacedRectSide\",\"uuid\":\"7acb360a-1230-4e27-92b8-6b3184352f22\"},{\"content\":{\"side\":\"RIGHT\"},\"type\":\"ConnectorPlacement.EquallySpacedRectSide\",\"uuid\":\"8c89d56c-1eb2-4c7c-8666-e0d9ca480c9b\"},{\"content\":{\"connectorIds\":[\"LConn1\"],\"side\":\"TOP\"},\"type\":\"ConnectorPlacement.EquallySpacedRectSide\",\"uuid\":\"50379f80-a646-4b72-9568-e30937a88a17\"}]},\"type\":\"ConnectorPlacement.EquallySpacedConnector\",\"uuid\":\"0fd64392-f5bf-42bb-9262-b488cfdbbdbf\"}],\"packageUris\":[\"http://schema.mathworks.com/mf0/Connector/R2020b\"],\"version\":\"1.0\"}"
  hanger_5_RIGID : Subsystem
  hanger_6_RIGID : Subsystem
  hanger_7_RIGID : Subsystem
  hanger_8_RIGID : Subsystem
  jetson_orin_nano_1_RIGID : Subsystem  Commented=on
  leg_1_RIGID : Subsystem
  leg_2_RIGID : Subsystem
  leg_joint_1_RIGID : Subsystem
      settings: PortSchema="{\"entries\":[{\"content\":{\"sides\":[{\"content\":{},\"type\":\"ConnectorPlacement.EquallySpacedRectSide\",\"uuid\":\"e4c68bcb-f3fe-4aba-8bbb-748bf6c2ba1e\"},{\"content\":{\"connectorIds\":[\"RConn1\"],\"side\":\"RIGHT\"},\"type\":\"ConnectorPlacement.EquallySpacedRectSide\",\"uuid\":\"1338b84e-cb3b-43ed-b934-4b64495642c6\"},{\"content\":{\"side\":\"TOP\"},\"type\":\"ConnectorPlacement.EquallySpacedRectSide\",\"uuid\":\"c07eb51d-104f-4d2f-bffb-19c5e8e904cd\"},{\"content\":{\"connectorIds\":[\"RConn2\"],\"side\":\"BOTTOM\"},\"type\":\"ConnectorPlacement.EquallySpacedRectSide\",\"uuid\":\"fc854f5d-a60f-47a0-b2a6-93c6d9c1db67\"}]},\"type\":\"ConnectorPlacement.EquallySpacedConnector\",\"uuid\":\"66267511-5957-447d-be6d-58b2f28344a3\"}],\"packageUris\":[\"http://schema.mathworks.com/mf0/Connector/R2020b\"],\"version\":\"1.0\"}"
  leg_joint_2_RIGID : Subsystem
      settings: PortSchema="{\"entries\":[{\"content\":{\"sides\":[{\"content\":{},\"type\":\"ConnectorPlacement.EquallySpacedRectSide\",\"uuid\":\"e4c68bcb-f3fe-4aba-8bbb-748bf6c2ba1e\"},{\"content\":{\"connectorIds\":[\"RConn1\"],\"side\":\"RIGHT\"},\"type\":\"ConnectorPlacement.EquallySpacedRectSide\",\"uuid\":\"1338b84e-cb3b-43ed-b934-4b64495642c6\"},{\"content\":{\"side\":\"TOP\"},\"type\":\"ConnectorPlacement.EquallySpacedRectSide\",\"uuid\":\"c07eb51d-104f-4d2f-bffb-19c5e8e904cd\"},{\"content\":{\"connectorIds\":[\"RConn2\"],\"side\":\"BOTTOM\"},\"type\":\"ConnectorPlacement.EquallySpacedRectSide\",\"uuid\":\"a008b5bd-ef4e-42cd-9cf4-6937e5bcfb2a\"}]},\"type\":\"ConnectorPlacement.EquallySpacedConnector\",\"uuid\":\"66267511-5957-447d-be6d-58b2f28344a3\"}],\"packageUris\":[\"http://schema.mathworks.com/mf0/Connector/R2020b\"],\"version\":\"1.0\"}"
  motor1 : Subsystem
  motor2 : Subsystem
  motor3 : Subsystem
  motor4 : Subsystem
  nylon_joint_1_RIGID : Subsystem
  nylon_joint_2_RIGID : Subsystem
  nylon_joint_3_RIGID : Subsystem
  nylon_joint_4_RIGID : Subsystem
  pixhawk6c_1_RIGID : Subsystem
      settings: PortSchema="{\"entries\":[{\"content\":{\"sides\":[{\"content\":{},\"type\":\"ConnectorPlacement.EquallySpacedRectSide\",\"uuid\":\"7acb360a-1230-4e27-92b8-6b3184352f22\"},{\"content\":{\"side\":\"RIGHT\"},\"type\":\"ConnectorPlacement.EquallySpacedRectSide\",\"uuid\":\"8c89d56c-1eb2-4c7c-8666-e0d9ca480c9b\"},{\"content\":{\"connectorIds\":[\"LConn1\"],\"side\":\"TOP\"},\"type\":\"ConnectorPlacement.EquallySpacedRectSide\",\"uuid\":\"50379f80-a646-4b72-9568-e30937a88a17\"}]},\"type\":\"ConnectorPlacement.EquallySpacedConnector\",\"uuid\":\"0fd64392-f5bf-42bb-9262-b488cfdbbdbf\"}],\"packageUris\":[\"http://schema.mathworks.com/mf0/Connector/R2020b\"],\"version\":\"1.0\"}"
  top_board_1_RIGID : Subsystem
      settings: PortSchema="{\"entries\":[{\"content\":{\"sides\":[{\"content\":{},\"type\":\"ConnectorPlacement.EquallySpacedRectSide\",\"uuid\":\"e4c68bcb-f3fe-4aba-8bbb-748bf6c2ba1e\"},{\"content\":{\"side\":\"RIGHT\"},\"type\":\"ConnectorPlacement.EquallySpacedRectSide\",\"uuid\":\"1338b84e-cb3b-43ed-b934-4b64495642c6\"},{\"content\":{\"connectorIds\":[\"LConn1\"],\"side\":\"TOP\"},\"type\":\"ConnectorPlacement.EquallySpacedRectSide\",\"uuid\":\"c07eb51d-104f-4d2f-bffb-19c5e8e904cd\"},{\"content\":{\"connectorIds\":[\"RConn1\"],\"side\":\"BOTTOM\"},\"type\":\"ConnectorPlacement.EquallySpacedRectSide\",\"uuid\":\"341ffeb0-a865-4b86-9c61-7f4d093e5d3a\"}]},\"type\":\"ConnectorPlacement.EquallySpacedConnector\",\"uuid\":\"66267511-5957-447d-be6d-58b2f28344a3\"}],\"packageUris\":[\"http://schema.mathworks.com/mf0/Connector/R2020b\"],\"version\":\"1.0\"}"
  F : PMIOPort  Side=Right
  F1 : PMIOPort  Port=2  Side=Right
  F2 : PMIOPort  Port=3  Side=Right
  F12 : PMIOPort  Port=4  Side=Left
  F3 : PMIOPort  Port=5  Side=Right
  connections:
  Turnigy_5000mAh_3S_1_RIGID/RConn1 -- bottom_board_1_RIGID/LConn2
  ankle_1_RIGID/RConn1 -- foot_1_RIGID/LConn1
  foam_4_RIGID/RConn1 -- foot_1_RIGID/LConn2
  motor1/LConn1 -- nylon_joint_3_RIGID/RConn1
  computer_board_1_RIGID/RConn2 -- hanger_5_RIGID/LConn1
  arm_1_RIGID/LConn1 -- arm_joint_1_RIGID/RConn1
  ankle_1_RIGID/LConn1 -- leg_1_RIGID/RConn1
  arm_joint_3_RIGID/LConn1 -- bottom_board_1_RIGID/RConn4
  bottom_board_1_RIGID/RConn7 -- hanger_4_RIGID/LConn1
  arm_joint_1_RIGID/LConn1 -- bottom_board_1_RIGID/RConn2
  leg_1_RIGID/LConn1 -- leg_joint_2_RIGID/RConn1
  motor4/LConn1 -- nylon_joint_1_RIGID/RConn1
  arm_4_RIGID/LConn1 -- arm_joint_2_RIGID/RConn1
  ankle_2_RIGID/RConn1 -- foot_2_RIGID/LConn1
  F3/RConn1 -- motor1/RConn1
  arm_2_RIGID/LConn1 -- arm_joint_3_RIGID/RConn1
  pixhawk6c_1_RIGID/LConn1 -- top_board_1_RIGID/RConn1
  bottom_board_1_RIGID/LConn1 -- hanger_2_RIGID/LConn1
  bottom_board_1_RIGID/LConn6 -- leg_joint_1_RIGID/RConn2
  bar_1_RIGID/LConn1 -- hanger_2_RIGID/RConn1
  computer_board_1_RIGID/LConn1 -- hanger_7_RIGID/RConn1
  foam_1_RIGID/LConn1 -- foot_1_RIGID/RConn1
  bar_2_RIGID/RConn2 -- hanger_1_RIGID/LConn1
  motor2/LConn1 -- nylon_joint_4_RIGID/RConn1
  ankle_2_RIGID/LConn1 -- leg_2_RIGID/RConn1
  motor3/LConn1 -- nylon_joint_2_RIGID/RConn1
  bottom_board_1_RIGID/LConn3 -- F12/RConn1
  computer_board_1_RIGID/RConn3 -- jetson_orin_nano_1_RIGID/LConn1
  arm_joint_2_RIGID/LConn1 -- bottom_board_1_RIGID/RConn1
  arm_1_RIGID/RConn1 -- nylon_joint_1_RIGID/LConn1
  bottom_board_1_RIGID/RConn6 -- hanger_3_RIGID/LConn1
  arm_4_RIGID/RConn1 -- nylon_joint_2_RIGID/LConn1
  bottom_board_1_RIGID/RConn5 -- top_board_1_RIGID/LConn1
  arm_3_RIGID/RConn1 -- nylon_joint_4_RIGID/LConn1
  bottom_board_1_RIGID/LConn4 -- hanger_1_RIGID/RConn1
  arm_2_RIGID/RConn1 -- nylon_joint_3_RIGID/LConn1
  bar_2_RIGID/RConn1 -- hanger_7_RIGID/LConn1
  computer_board_1_RIGID/LConn2 -- hanger_8_RIGID/LConn1
  F/RConn1 -- motor3/RConn1
  F2/RConn1 -- motor2/RConn1
  computer_board_1_RIGID/RConn1 -- hanger_6_RIGID/LConn1
  foam_2_RIGID/RConn1 -- foot_2_RIGID/LConn2
  bottom_board_1_RIGID/LConn5 -- leg_joint_2_RIGID/RConn2
  foam_3_RIGID/LConn1 -- foot_2_RIGID/RConn1
  arm_joint_4_RIGID/LConn1 -- bottom_board_1_RIGID/RConn3
  leg_2_RIGID/LConn1 -- leg_joint_1_RIGID/RConn1
  arm_3_RIGID/LConn1 -- arm_joint_4_RIGID/RConn1
  F1/RConn1 -- motor4/RConn1

== system quad_CAD_asgsm/Plant Quadcopter/prop1 ==
  ReferenceFrame : sm_lib/Frames and Transforms/Reference Frame
  Solid : sm_lib/Body Elements/File Solid  ExtGeomFileName=propeller_Predeterminado_sldprt.STEP  UnitType=FromFile  ExtGeomFileUnits=m  StepReaderType=HEX  ExportConvexHullGeometry=off  InertiaType=Custom  BasedOnType=DensityFromFile  Density=1000  DensityUnits=kg/m^3  Mass=smiData.Solid(11).mass  MassUnits=kg  CenterOfMass=smiData.Solid(11).CoM  CenterOfMassUnits=mm  MomentsOfInertia=smiData.Solid(11).MoI  MomentsOfInertiaUnits=kg*mm^2  ProductsOfInertia=smiData.Solid(11).PoI  ProductsOfInertiaUnits=kg*mm^2  GraphicType=FromGeometry  MarkerShape=Sphere  MarkerSize=10  GraphicVisPropType=SimpleVisualProperties  GraphicDiffuseColor=smiData.Solid(11).color  GraphicOpacity=smiData.Solid(11).opacity  GraphicSpecularColor=[0.5 0.5 0.5 1.0]  GraphicAmbientColor=[0.15 0.15 0.15 1.0]  GraphicEmissiveColor=[0.0 0.0 0.0 1.0]  GraphicShininess=75  DoExposeReferenceFrame=on  SerializedFrames=<Frames/>
  Transform : sm_lib/Frames and Transforms/Rigid Transform  RotationMethod=ArbitraryAxis  FollAlignAxisA=+X  BaseAlignAxisA=+Y  FollAlignAxisB=+Y  BaseAlignAxisB=+Z  RotationStandardAxis=+Z  RotationAngle=smiData.RigidTransform(12).angle  RotationAngleUnits=rad  RotationArbitraryAxis=smiData.RigidTransform(12).axis  RotationSequenceAxes=FollowerAxes  RotationSequence=XYX  RotationSequenceAngles=[0 0 0]  RotationSequenceAnglesUnits=deg  RotationMatrix=[1 0 0;0 1 0;0 0 1]  Quaternion=[1 0 0 0]  TranslationMethod=Cartesian  TranslationCartesianOffset=smiData.RigidTransform(12).translation  TranslationCartesianOffsetUnits=mm  TranslationStandardAxis=+Z  TranslationStandardOffset=0  TranslationStandardOffsetUnits=m  TranslationROffset=0  TranslationROffsetUnits=m  TranslationThetaOffset=0  TranslationThetaOffsetUnits=deg  TranslationZOffset=0  TranslationZOffsetUnits=m
  F : PMIOPort  Side=Left
  connections:
  Solid/RConn1 -- ReferenceFrame/RConn1 -- Transform/LConn1
  Transform/RConn1 -- F/RConn1

== system quad_CAD_asgsm/Plant Quadcopter/prop2 ==
  ReferenceFrame : sm_lib/Frames and Transforms/Reference Frame
  Solid : sm_lib/Body Elements/File Solid  ExtGeomFileName=propeller_Predeterminado_sldprt.STEP  UnitType=FromFile  ExtGeomFileUnits=m  StepReaderType=HEX  ExportConvexHullGeometry=off  InertiaType=Custom  BasedOnType=DensityFromFile  Density=1000  DensityUnits=kg/m^3  Mass=smiData.Solid(11).mass  MassUnits=kg  CenterOfMass=smiData.Solid(11).CoM  CenterOfMassUnits=mm  MomentsOfInertia=smiData.Solid(11).MoI  MomentsOfInertiaUnits=kg*mm^2  ProductsOfInertia=smiData.Solid(11).PoI  ProductsOfInertiaUnits=kg*mm^2  GraphicType=FromGeometry  MarkerShape=Sphere  MarkerSize=10  GraphicVisPropType=SimpleVisualProperties  GraphicDiffuseColor=smiData.Solid(11).color  GraphicOpacity=smiData.Solid(11).opacity  GraphicSpecularColor=[0.5 0.5 0.5 1.0]  GraphicAmbientColor=[0.15 0.15 0.15 1.0]  GraphicEmissiveColor=[0.0 0.0 0.0 1.0]  GraphicShininess=75  DoExposeReferenceFrame=on  SerializedFrames=<Frames/>
  Transform : sm_lib/Frames and Transforms/Rigid Transform  RotationMethod=ArbitraryAxis  FollAlignAxisA=+X  BaseAlignAxisA=+Y  FollAlignAxisB=+Y  BaseAlignAxisB=+Z  RotationStandardAxis=+Z  RotationAngle=smiData.RigidTransform(18).angle  RotationAngleUnits=rad  RotationArbitraryAxis=smiData.RigidTransform(18).axis  RotationSequenceAxes=FollowerAxes  RotationSequence=XYX  RotationSequenceAngles=[0 0 0]  RotationSequenceAnglesUnits=deg  RotationMatrix=[1 0 0;0 1 0;0 0 1]  Quaternion=[1 0 0 0]  TranslationMethod=Cartesian  TranslationCartesianOffset=smiData.RigidTransform(18).translation  TranslationCartesianOffsetUnits=mm  TranslationStandardAxis=+Z  TranslationStandardOffset=0  TranslationStandardOffsetUnits=m  TranslationROffset=0  TranslationROffsetUnits=m  TranslationThetaOffset=0  TranslationThetaOffsetUnits=deg  TranslationZOffset=0  TranslationZOffsetUnits=m
  F : PMIOPort  Side=Left
  connections:
  Solid/RConn1 -- ReferenceFrame/RConn1 -- Transform/LConn1
  Transform/RConn1 -- F/RConn1

== system quad_CAD_asgsm/Plant Quadcopter/prop3 ==
  ReferenceFrame : sm_lib/Frames and Transforms/Reference Frame
  Solid : sm_lib/Body Elements/File Solid  ExtGeomFileName=propeller_Predeterminado_sldprt.STEP  UnitType=FromFile  ExtGeomFileUnits=m  StepReaderType=HEX  ExportConvexHullGeometry=off  InertiaType=Custom  BasedOnType=DensityFromFile  Density=1000  DensityUnits=kg/m^3  Mass=smiData.Solid(11).mass  MassUnits=kg  CenterOfMass=smiData.Solid(11).CoM  CenterOfMassUnits=mm  MomentsOfInertia=smiData.Solid(11).MoI  MomentsOfInertiaUnits=kg*mm^2  ProductsOfInertia=smiData.Solid(11).PoI  ProductsOfInertiaUnits=kg*mm^2  GraphicType=FromGeometry  MarkerShape=Sphere  MarkerSize=10  GraphicVisPropType=SimpleVisualProperties  GraphicDiffuseColor=smiData.Solid(11).color  GraphicOpacity=smiData.Solid(11).opacity  GraphicSpecularColor=[0.5 0.5 0.5 1.0]  GraphicAmbientColor=[0.15 0.15 0.15 1.0]  GraphicEmissiveColor=[0.0 0.0 0.0 1.0]  GraphicShininess=75  DoExposeReferenceFrame=on  SerializedFrames=<Frames/>
  Transform : sm_lib/Frames and Transforms/Rigid Transform  RotationMethod=ArbitraryAxis  FollAlignAxisA=+X  BaseAlignAxisA=+Y  FollAlignAxisB=+Y  BaseAlignAxisB=+Z  RotationStandardAxis=+Z  RotationAngle=smiData.RigidTransform(16).angle  RotationAngleUnits=rad  RotationArbitraryAxis=smiData.RigidTransform(16).axis  RotationSequenceAxes=FollowerAxes  RotationSequence=XYX  RotationSequenceAngles=[0 0 0]  RotationSequenceAnglesUnits=deg  RotationMatrix=[1 0 0;0 1 0;0 0 1]  Quaternion=[1 0 0 0]  TranslationMethod=Cartesian  TranslationCartesianOffset=smiData.RigidTransform(16).translation  TranslationCartesianOffsetUnits=mm  TranslationStandardAxis=+Z  TranslationStandardOffset=0  TranslationStandardOffsetUnits=m  TranslationROffset=0  TranslationROffsetUnits=m  TranslationThetaOffset=0  TranslationThetaOffsetUnits=deg  TranslationZOffset=0  TranslationZOffsetUnits=m
  F : PMIOPort  Side=Left
  connections:
  Solid/RConn1 -- ReferenceFrame/RConn1 -- Transform/LConn1
  Transform/RConn1 -- F/RConn1

== system quad_CAD_asgsm/Plant Quadcopter/prop4 ==
  ReferenceFrame : sm_lib/Frames and Transforms/Reference Frame
  Solid : sm_lib/Body Elements/File Solid  ExtGeomFileName=propeller_Predeterminado_sldprt.STEP  UnitType=FromFile  ExtGeomFileUnits=m  StepReaderType=HEX  ExportConvexHullGeometry=off  InertiaType=Custom  BasedOnType=DensityFromFile  Density=1000  DensityUnits=kg/m^3  Mass=smiData.Solid(11).mass  MassUnits=kg  CenterOfMass=smiData.Solid(11).CoM  CenterOfMassUnits=mm  MomentsOfInertia=smiData.Solid(11).MoI  MomentsOfInertiaUnits=kg*mm^2  ProductsOfInertia=smiData.Solid(11).PoI  ProductsOfInertiaUnits=kg*mm^2  GraphicType=FromGeometry  MarkerShape=Sphere  MarkerSize=10  GraphicVisPropType=SimpleVisualProperties  GraphicDiffuseColor=smiData.Solid(11).color  GraphicOpacity=smiData.Solid(11).opacity  GraphicSpecularColor=[0.5 0.5 0.5 1.0]  GraphicAmbientColor=[0.15 0.15 0.15 1.0]  GraphicEmissiveColor=[0.0 0.0 0.0 1.0]  GraphicShininess=75  DoExposeReferenceFrame=on  SerializedFrames=<Frames/>
  Transform : sm_lib/Frames and Transforms/Rigid Transform  RotationMethod=ArbitraryAxis  FollAlignAxisA=+X  BaseAlignAxisA=+Y  FollAlignAxisB=+Y  BaseAlignAxisB=+Z  RotationStandardAxis=+Z  RotationAngle=smiData.RigidTransform(14).angle  RotationAngleUnits=rad  RotationArbitraryAxis=smiData.RigidTransform(14).axis  RotationSequenceAxes=FollowerAxes  RotationSequence=XYX  RotationSequenceAngles=[0 0 0]  RotationSequenceAnglesUnits=deg  RotationMatrix=[1 0 0;0 1 0;0 0 1]  Quaternion=[1 0 0 0]  TranslationMethod=Cartesian  TranslationCartesianOffset=smiData.RigidTransform(14).translation  TranslationCartesianOffsetUnits=mm  TranslationStandardAxis=+Z  TranslationStandardOffset=0  TranslationStandardOffsetUnits=m  TranslationROffset=0  TranslationROffsetUnits=m  TranslationThetaOffset=0  TranslationThetaOffsetUnits=deg  TranslationZOffset=0  TranslationZOffsetUnits=m
  F : PMIOPort  Side=Left
  connections:
  Solid/RConn1 -- ReferenceFrame/RConn1 -- Transform/LConn1
  Transform/RConn1 -- F/RConn1

== system quad_CAD_asgsm/Trajectory/Kronecker product3 ==
  q : Inport
  p : Inport  Port=2
  Kronecker_product : MATLAB Function  TreatAsAtomicUnit=on
  r : Outport
  wires:
  q/1 -> Kronecker_product/1(q)
  p/1 -> Kronecker_product/2(p)
  Kronecker_product/1(r) -> r/1

== system quad_CAD_asgsm/Trajectory/Kronecker product5 ==
  q : Inport
  p : Inport  Port=2
  Kronecker_product : MATLAB Function  TreatAsAtomicUnit=on
  r : Outport
  wires:
  q/1 -> Kronecker_product/1(q)
  p/1 -> Kronecker_product/2(p)
  Kronecker_product/1(r) -> r/1

== system quad_CAD_asgsm/Plant Quadcopter/Quad Simscape/Turnigy_5000mAh_3S_1_RIGID ==
  ReferenceFrame : sm_lib/Frames and Transforms/Reference Frame
  Solid : sm_lib/Body Elements/File Solid  ExtGeomFileName=Turnigy 5000mAh 3S_Predeterminado_sldprt.STEP  UnitType=FromFile  ExtGeomFileUnits=m  StepReaderType=HEX  ExportConvexHullGeometry=off  InertiaType=Custom  BasedOnType=DensityFromFile  Density=1000  DensityUnits=kg/m^3  Mass=smiData.Solid(17).mass  MassUnits=kg  CenterOfMass=smiData.Solid(17).CoM  CenterOfMassUnits=mm  MomentsOfInertia=smiData.Solid(17).MoI  MomentsOfInertiaUnits=kg*mm^2  ProductsOfInertia=smiData.Solid(17).PoI  ProductsOfInertiaUnits=kg*mm^2  GraphicType=FromGeometry  MarkerShape=Sphere  MarkerSize=10  GraphicVisPropType=SimpleVisualProperties  GraphicDiffuseColor=smiData.Solid(17).color  GraphicOpacity=smiData.Solid(17).opacity  GraphicSpecularColor=[0.5 0.5 0.5 1.0]  GraphicAmbientColor=[0.15 0.15 0.15 1.0]  GraphicEmissiveColor=[0.0 0.0 0.0 1.0]  GraphicShininess=75  DoExposeReferenceFrame=on  SerializedFrames=<Frames/>
  Transform : sm_lib/Frames and Transforms/Rigid Transform  RotationMethod=ArbitraryAxis  FollAlignAxisA=+X  BaseAlignAxisA=+Y  FollAlignAxisB=+Y  BaseAlignAxisB=+Z  RotationStandardAxis=+Z  RotationAngle=smiData.RigidTransform(38).angle  RotationAngleUnits=rad  RotationArbitraryAxis=smiData.RigidTransform(38).axis  RotationSequenceAxes=FollowerAxes  RotationSequence=XYX  RotationSequenceAngles=[0 0 0]  RotationSequenceAnglesUnits=deg  RotationMatrix=[1 0 0;0 1 0;0 0 1]  Quaternion=[1 0 0 0]  TranslationMethod=Cartesian  TranslationCartesianOffset=smiData.RigidTransform(38).translation  TranslationCartesianOffsetUnits=mm  TranslationStandardAxis=+Z  TranslationStandardOffset=0  TranslationStandardOffsetUnits=m  TranslationROffset=0  TranslationROffsetUnits=m  TranslationThetaOffset=0  TranslationThetaOffsetUnits=deg  TranslationZOffset=0  TranslationZOffsetUnits=m
  F : PMIOPort  Side=Right
  connections:
  Solid/RConn1 -- ReferenceFrame/RConn1 -- Transform/LConn1
  Transform/RConn1 -- F/RConn1
